simulink model "sim_env_falling_leaf"  (R2023b)
settings: Solver=ode113  StartTime=0.0  StopTime=50  RelTol=1e-3
model workspace (MAT data in the model file):
  ail_0 = -0.0765
settings Model: PauseTimes=25  Creator=ac140857  LastModifiedBy=fabioschneider
settings DebuggingCC: AlgebraicLoopMsg=none  ModelReferenceExtraNoncontSigs=none

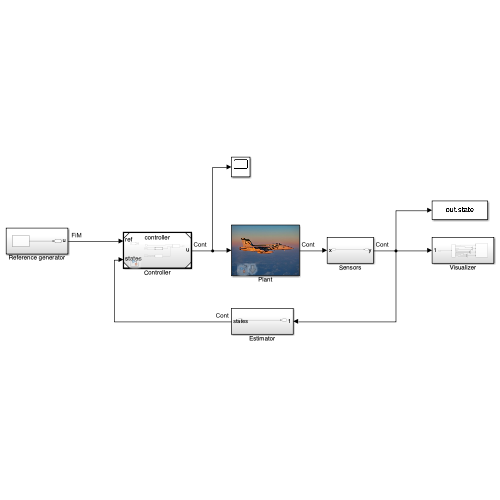
[thumbnail: Simulink's stored preview of the top-level diagram]
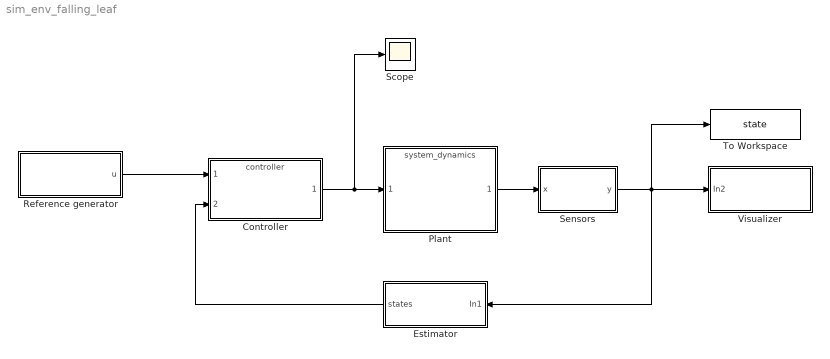
== system sim_env_falling_leaf ==
  Controller : ModelReference  ModelNameDialog=controller.slx  SimulationMode=Normal  ModelReferenceVersion=1.6
  Estimator : Subsystem
  Plant : ModelReference  ModelNameDialog=system_dynamics.slx  SimulationMode=Normal  ModelReferenceVersion=4.91
      mask Display: image('F-18_image Small.jpeg');
  Reference generator : Subsystem
  Scope : Scope
  Sensors : Subsystem
  To Workspace : ToWorkspace  VariableName=state  SaveFormat=Timeseries  SampleTime=-1
  Visualizer : Subsystem
  wires:
  Reference generator/1(u) -> Controller/1
  Estimator/1(states) -> Controller/2
  Sensors/1(y) -> To Workspace/1, Visualizer/1(In2), Estimator/1(In1)
  Controller/1 -> Scope/1, Plant/1
  Plant/1 -> Sensors/1(x)

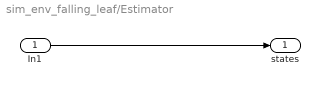
== system sim_env_falling_leaf/Estimator ==
  In1 : Inport
  states : Outport
  wires:
  In1/1 -> states/1

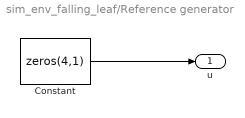
== system sim_env_falling_leaf/Reference generator ==
  Constant : Constant  Value=zeros(4,1)  SampleTime=-1
  u : Outport
  wires:
  Constant/1 -> u/1

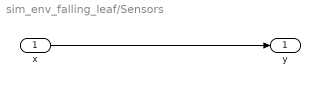
== system sim_env_falling_leaf/Sensors ==
  x : Inport
  y : Outport
  wires:
  x/1 -> y/1

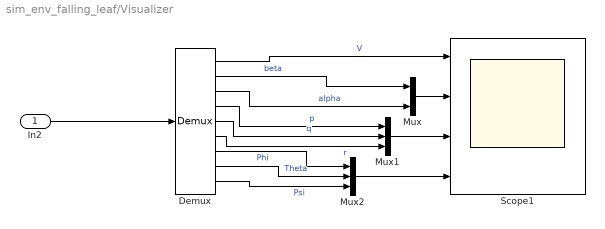
== system sim_env_falling_leaf/Visualizer ==
  In2 : Inport
  Demux : Demux  Outputs=9
  Mux : Mux  Inputs=2
  Mux1 : Mux  Inputs=3
  Mux2 : Mux  Inputs=3
  Scope1 : Scope  NumInputPorts=4
  wires:
  In2/1 -> Demux/1
  Demux/6 -> Mux1/3  "r"
  Demux/5 -> Mux1/2  "q"
  Demux/4 -> Mux1/1  "p"
  Demux/8 -> Mux2/2  "Theta"
  Demux/7 -> Mux2/1  "Phi"
  Demux/2 -> Mux/1  "beta"
  Demux/1 -> Scope1/1  "V"
  Mux/1 -> Scope1/2
  Demux/3 -> Mux/2  "alpha"
  Mux2/1 -> Scope1/4
  Demux/9 -> Mux2/3  "Psi"
  Mux1/1 -> Scope1/3
